simulink model "PLL_complete"  (Simulink 7.7)
settings: Solver=ode45  StartTime=0.0  StopTime=simtime  RelTol=1e-3
values from neighbouring files (symbols this model uses):
  cycles = input('\nNo. of cycles to be observed per change: ')    [PLL_Init_complete.m]
  fq_step = input('Frequency step observed (indicate +/-) (Hz): ')    [PLL_Init_complete.m]
  k = sqrt(2)    [PLL_Init_complete.m]
  ki = (wn^2)/Em    [PLL_Init_complete.m]    (also in plot3D_selfconsistent_cardan_complete.m)
  kp = 2*del*wn/Em    [PLL_Init_complete.m]    (also in plot3D_selfconsistent_cardan_complete.m)
  ph_jump = input('Phase jump observed (indicate +/-) (rad): ')    [PLL_Init_complete.m]
  Ts = 0.1e-3    (= 0.0001)    [PLL_Init_complete.m]
  wc = 2*pi*50    (= 314.159265359)    [PLL_Init_complete.m]
  wf = 2*pi*50/sqrt(2)    [PLL_Init_complete.m]
libraries: aerolibobsolete x7
settings Model: Creator=pradhyumna  LastModifiedBy=Sambhav

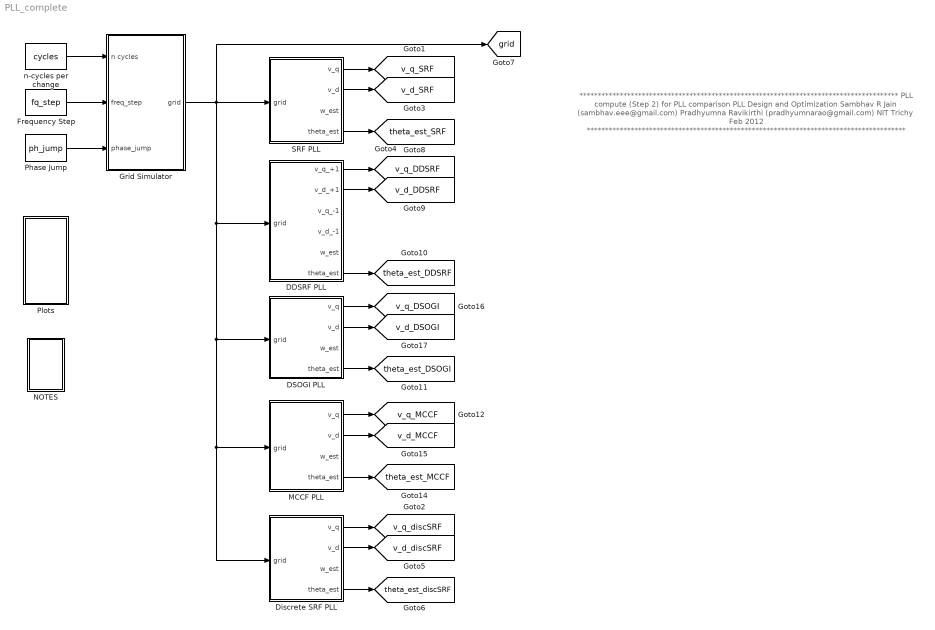
== system PLL_complete ==
  note: ***************************************************************************************
      | PLL compute (Step 2) for PLL comparison
      |
      | PLL Design and Optimization
      |
      | Sambhav R Jain (sambhav.eee@gmail.com)
      | Pradhyumna Ravikirthi (pradhyumnarao@gmail.com)
      | NIT Trichy
      | Feb 2012
      |
      | ***************************************************************************************
  DDSRF PLL : Subsystem
  DSOGI PLL : Subsystem
  Discrete SRF PLL : Subsystem
  Frequency Step : Constant  Value=fq_step
  Grid Simulator : Subsystem
  MCCF PLL : Subsystem
  NOTES : Subsystem
  Phase Jump : Constant  Value=ph_jump
  Plots : Subsystem
  SRF PLL : Subsystem
  n-cycles per change : Constant  Value=cycles
  tag scope: grid=global, theta_est_DDSRF=global, theta_est_DSOGI=global, theta_est_MCCF=global, theta_est_SRF=global, theta_est_discSRF=global, v_d_DDSRF=global, v_d_DSOGI=global, v_d_MCCF=global, v_d_SRF=global, v_d_discSRF=global, v_q_DDSRF=global, v_q_DSOGI=global, v_q_MCCF=global, v_q_SRF=global, v_q_discSRF=global
  wires:
  SRF PLL/1(v_q) -> [v_q_SRF]
  SRF PLL/2(v_d) -> [v_d_SRF]
  SRF PLL/4(theta_est) -> [theta_est_SRF]
  DDSRF PLL/1(v_q_+1) -> [v_q_DDSRF]
  DDSRF PLL/2(v_d_+1) -> [v_d_DDSRF]
  DDSRF PLL/6(theta_est) -> [theta_est_DDSRF]
  DSOGI PLL/1(v_q) -> [v_q_DSOGI]
  DSOGI PLL/2(v_d) -> [v_d_DSOGI]
  DSOGI PLL/4(theta_est) -> [theta_est_DSOGI]
  MCCF PLL/1(v_q) -> [v_q_MCCF]
  MCCF PLL/2(v_d) -> [v_d_MCCF]
  MCCF PLL/4(theta_est) -> [theta_est_MCCF]
  Discrete SRF PLL/1(v_q) -> [v_q_discSRF]
  Discrete SRF PLL/2(v_d) -> [v_d_discSRF]
  Discrete SRF PLL/4(theta_est) -> [theta_est_discSRF]
  n-cycles per change/1 -> Grid Simulator/1(n cycles)
  Frequency Step/1 -> Grid Simulator/2(freq_step)
  Phase Jump/1 -> Grid Simulator/3(phase_jump)
  Grid Simulator/1(grid) -> SRF PLL/1(grid), DDSRF PLL/1(grid), DSOGI PLL/1(grid), MCCF PLL/1(grid), Discrete SRF PLL/1(grid), [grid]

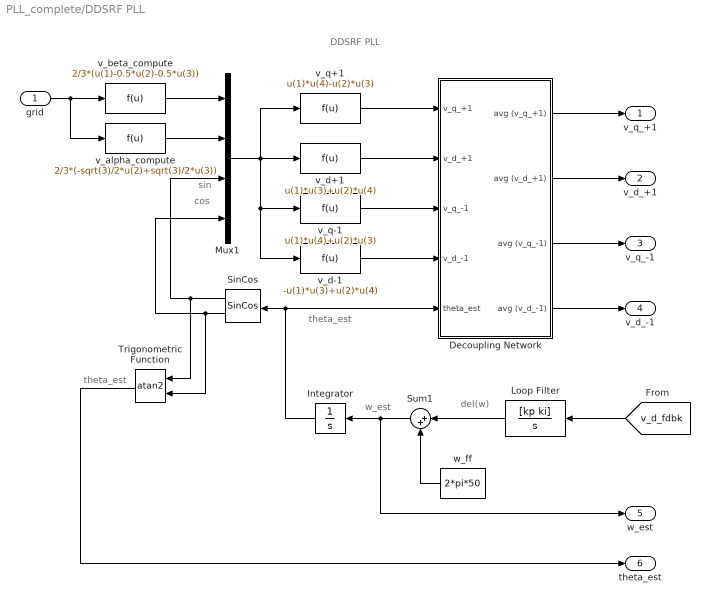
== system PLL_complete/DDSRF PLL ==
  note: cos
  note: sin
  note: del(w)
  note: w_est
  note: theta_est
  note: DDSRF PLL
  note: theta_est
  grid : Inport
  Decoupling Network : Subsystem
  Integrator : Integrator
  Loop Filter : TransferFcn  Numerator=[kp ki]  Denominator=[1 0]
  Mux1 : Mux
  SinCos : aerolibobsolete/SinCos  SystemSampleTime=-1
  Sum1 : Sum  Inputs=|++
  Trigonometric Function : Trigonometry  Operator=atan2
  v_alpha_compute : Fcn  Expr=2/3*(-sqrt(3)/2*u(2)+sqrt(3)/2*u(3))
  v_beta_compute : Fcn  Expr=2/3*(u(1)-0.5*u(2)-0.5*u(3))
  v_d+1 : Fcn  Expr=u(1)*u(3)+u(2)*u(4)
  v_d-1 : Fcn  Expr=-u(1)*u(3)+u(2)*u(4)
  v_q+1 : Fcn  Expr=u(1)*u(4)-u(2)*u(3)
  v_q-1 : Fcn  Expr=u(1)*u(4)+u(2)*u(3)
  w_ff : Constant  Value=2*pi*50
  v_q_+1 : Outport
  v_d_+1 : Outport  Port=2
  v_q_-1 : Outport  Port=3
  v_d_-1 : Outport  Port=4
  w_est : Outport  Port=5
  theta_est : Outport  Port=6
  wires:
  SinCos/2 -> Mux1/4, Trigonometric Function/2
  SinCos/1 -> Mux1/3, Trigonometric Function/1
  v_alpha_compute/1 -> Mux1/2
  v_beta_compute/1 -> Mux1/1
  v_q+1/1 -> Decoupling Network/1(v_q_+1)
  v_d+1/1 -> Decoupling Network/2(v_d_+1)
  v_q-1/1 -> Decoupling Network/3(v_q_-1)
  v_d-1/1 -> Decoupling Network/4(v_d_-1)
  Mux1/1 -> v_d+1/1, v_q+1/1, v_q-1/1, v_d-1/1
  Loop Filter/1 -> Sum1/1
  Sum1/1 -> Integrator/1, w_est/1
  w_ff/1 -> Sum1/2
  Decoupling Network/2(avg (v_d_+1)) -> v_d_+1/1
  Integrator/1 -> SinCos/1, Decoupling Network/5(theta_est)
  grid/1 -> v_beta_compute/1, v_alpha_compute/1
  Decoupling Network/1(avg (v_q_+1)) -> v_q_+1/1
  Trigonometric Function/1 -> theta_est/1
  Decoupling Network/3(avg (v_q_-1)) -> v_q_-1/1
  Decoupling Network/4(avg (v_d_-1)) -> v_d_-1/1
  [v_d_fdbk] -> Loop Filter/1

== system PLL_complete/DSOGI PLL ==
  note: check it out for k = 0.1 !!!!
      | sluggish response
  note: DSOGI PLL
  grid : Inport
  Gain : Gain  Gain=1/2
  Gain1 : Gain  Gain=1/2
  SOGI - alpha : Subsystem
  SOGI - beta : Subsystem
  SRFPLL : Subsystem
  Saturation : Saturate  UpperLimit=2*pi*60  LowerLimit=2*pi*40
  Sum : Sum  Inputs=|++
  Sum1 : Sum  Inputs=|-+
  to reduce  sampling rate of SRF PLL : Gain  SampleTime=0.01
  v_alpha_compute : Fcn  Expr=2/3*(-sqrt(3)/2*u(2)+sqrt(3)/2*u(3))
  v_beta_compute : Fcn  Expr=2/3*(u(1)-0.5*u(2)-0.5*u(3))
  v_q : Outport
  v_d : Outport  Port=2
  w_est : Outport  Port=3
  theta_est : Outport  Port=4
  tag scope: w_est_DSOGI=global
  wires:
  v_alpha_compute/1 -> SOGI - alpha/1(v_alpha)
  v_beta_compute/1 -> SOGI - beta/1(v_beta)
  grid/1 -> v_alpha_compute/1, v_beta_compute/1
  SOGI - beta/1(v_beta_dash) -> Sum/1
  SOGI - alpha/2(q_v_alpha_dash) -> Sum/2
  SOGI - beta/2(q_v_beta_dash) -> Sum1/1
  SOGI - alpha/1(v_alpha_dash) -> Sum1/2
  Sum/1 -> Gain/1
  Gain/1 -> SRFPLL/1(v_beta_1+)
  Sum1/1 -> Gain1/1
  to reduce  sampling rate of SRF PLL/1 -> Saturation/1
  Saturation/1 -> [w_est_DSOGI]
  SRFPLL/4(w_est) -> to reduce  sampling rate of SRF PLL/1, w_est/1
  SRFPLL/1(V_q_space_vector) -> v_q/1
  SRFPLL/2(V_d_error) -> v_d/1
  SRFPLL/3(theta_est) -> theta_est/1
  Gain1/1 -> SRFPLL/2(v_alpha_1+)

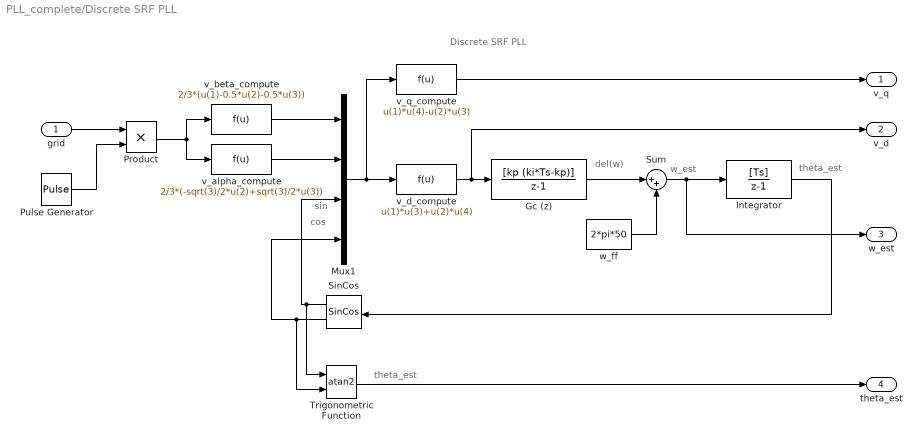
== system PLL_complete/Discrete SRF PLL ==
  note: theta_est
  note: w_est
  note: del(w)
  note: theta_est
  note: Discrete SRF PLL
  note: cos
  note: sin
  grid : Inport
  Gc (z) : DiscreteTransferFcn  Numerator=[kp (ki*Ts-kp)]  Denominator=[1 -1]  SampleTime=0.0001
  Integrator : DiscreteTransferFcn  Numerator=[Ts]  Denominator=[1 -1]  SampleTime=0.0001
  Mux1 : Mux
  Product : Product  RndMeth=Zero
  Pulse Generator : DiscretePulseGenerator  PulseType=Time based  Period=Ts  PulseWidth=10
  SinCos : aerolibobsolete/SinCos  SystemSampleTime=-1
  Sum : Sum  Inputs=|++
  Trigonometric Function : Trigonometry  Operator=atan2
  v_alpha_compute : Fcn  Expr=2/3*(-sqrt(3)/2*u(2)+sqrt(3)/2*u(3))
  v_beta_compute : Fcn  Expr=2/3*(u(1)-0.5*u(2)-0.5*u(3))
  v_d_compute : Fcn  Expr=u(1)*u(3)+u(2)*u(4)
  v_q_compute : Fcn  Expr=u(1)*u(4)-u(2)*u(3)
  w_ff : Constant  Value=2*pi*50
  v_q : Outport
  v_d : Outport  Port=2
  w_est : Outport  Port=3
  theta_est : Outport  Port=4
  wires:
  Trigonometric Function/1 -> theta_est/1
  v_q_compute/1 -> v_q/1
  w_ff/1 -> Sum/2
  v_beta_compute/1 -> Mux1/1
  v_alpha_compute/1 -> Mux1/2
  SinCos/1 -> Trigonometric Function/1, Mux1/3
  SinCos/2 -> Trigonometric Function/2, Mux1/4
  Mux1/1 -> v_q_compute/1, v_d_compute/1
  v_d_compute/1 -> v_d/1, Gc (z)/1
  Sum/1 -> w_est/1, Integrator/1
  Gc (z)/1 -> Sum/1
  Integrator/1 -> SinCos/1
  Pulse Generator/1 -> Product/2
  Product/1 -> v_beta_compute/1, v_alpha_compute/1
  grid/1 -> Product/1

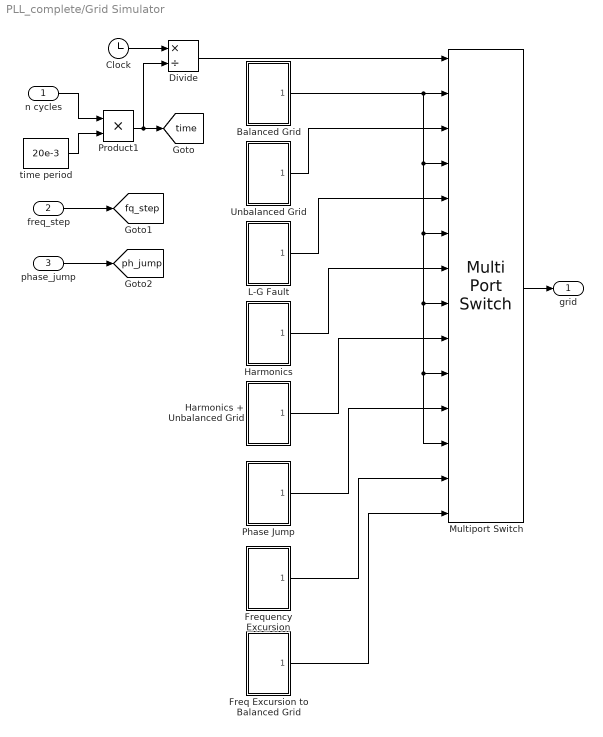
== system PLL_complete/Grid Simulator ==
  n cycles : Inport
  freq_step : Inport  Port=2
  phase_jump : Inport  Port=3
  Balanced Grid : Subsystem
  Clock : Clock
  Divide : Product  Inputs=*/
  Freq Excursion to Balanced Grid : Subsystem
  Frequency Excursion : Subsystem
  Harmonics : Subsystem
  Harmonics + Unbalanced Grid : Subsystem
  L-G Fault : Subsystem
  Multiport Switch : MultiPortSwitch  Inputs=13  DiagnosticForDefault=None  zeroidx=off
  Phase Jump : Subsystem
  Product1 : Product  RndMeth=Zero
  Unbalanced Grid : Subsystem
  time period : Constant  Value=20e-3
  grid : Outport
  tag scope: fq_step=global, ph_jump=global, time=global
  wires:
  Clock/1 -> Divide/1
  time period/1 -> Product1/2
  Product1/1 -> Divide/2, [time]
  Divide/1 -> Multiport Switch/1
  n cycles/1 -> Product1/1
  Multiport Switch/1 -> grid/1
  freq_step/1 -> [fq_step]
  Balanced Grid/1(v_grid) -> Multiport Switch/2, Multiport Switch/4, Multiport Switch/6, Multiport Switch/8, Multiport Switch/10, Multiport Switch/12
  Unbalanced Grid/1(v_grid) -> Multiport Switch/3
  L-G Fault/1(v_grid) -> Multiport Switch/5
  Harmonics/1(v_grid) -> Multiport Switch/7
  Harmonics + Unbalanced Grid/1(v_grid) -> Multiport Switch/9
  phase_jump/1 -> [ph_jump]
  Phase Jump/1(v_grid) -> Multiport Switch/11
  Frequency Excursion/1(v_grid) -> Multiport Switch/13
  Freq Excursion to Balanced Grid/1(v_grid) -> Multiport Switch/14

== system PLL_complete/MCCF PLL ==
  note: MCCF PLL
  grid : Inport
  MCCF module : Subsystem
  SRFPLL : Subsystem
  Saturation : Saturate  UpperLimit=2*pi*60  LowerLimit=2*pi*40
  to reduce  sampling rate of SRF PLL : Gain  SampleTime=0.01
  v_alpha_compute : Fcn  Expr=2/3*(-sqrt(3)/2*u(2)+sqrt(3)/2*u(3))
  v_beta_compute : Fcn  Expr=2/3*(u(1)-0.5*u(2)-0.5*u(3))
  v_q : Outport
  v_d : Outport  Port=2
  w_est : Outport  Port=3
  theta_est : Outport  Port=4
  tag scope: w_est_MCCF=global
  wires:
  v_alpha_compute/1 -> MCCF module/2(v_alpha)
  v_beta_compute/1 -> MCCF module/1(v_beta)
  MCCF module/1(v_beta_est_1+) -> SRFPLL/1(v_beta_1+)
  MCCF module/2(v_alpha_est_1+) -> SRFPLL/2(v_alpha_1+)
  to reduce  sampling rate of SRF PLL/1 -> Saturation/1
  Saturation/1 -> [w_est_MCCF]
  SRFPLL/4(w_est) -> to reduce  sampling rate of SRF PLL/1, w_est/1
  grid/1 -> v_beta_compute/1, v_alpha_compute/1
  SRFPLL/1(V_q_space_vector) -> v_q/1
  SRFPLL/2(V_d_error) -> v_d/1
  SRFPLL/3(theta_est) -> theta_est/1

== system PLL_complete/NOTES ==
  note: T = 0:002247
  note: ki = kp/T
  note: kp = -2.85
  note: Em = - Vm = - 230 * sqrt ( 2 )
      | del = - ( kp / 2 ) * sqrt ( Em / ki )
      | wn = sqrt ( ki * Em )
      | ki = kp / T
  note: Design of kp, ki
      |
      | ki = wn^2 / Em
      | kp = - 2 * del * sqrt ( ki / Em )
      | Weiner Method
      | (for optimum performance)
      | del = 1 / sqrt ( 2 )
  note: Calculated values
      |
      | del = 1 / sqrt ( 2 )
      | wn = 2 * pi * 100
      | ki = - 1213.7
      | kp = - 2.7318
  note: k = 1/sqrt(2) = wf/w
  note: wf = 2*pi*50*k
  note: kp = -20
  note: ki = - 246.7000
  note: Not sure about the loop filter design
  note: DDSRF
  note: k = sqrt(2) ----> optimum performance
  note: DSOGI
  note: MCCF
      | wc = 2*pi*50
  note: plot(time(3500:6500),v_q(3500:6500,:))
  note: k = 0.1 ------> sluggish, but harmonics are dealt well
  note: kp, ki same as DDSRF
  note: k = 1/sqrt(2) = wf/w
  note: wf = 2*pi*50*k
  note: kp = -20
  note: ki = - 246.7000
  note: Not sure about the loop filter design
  note: DDSRF

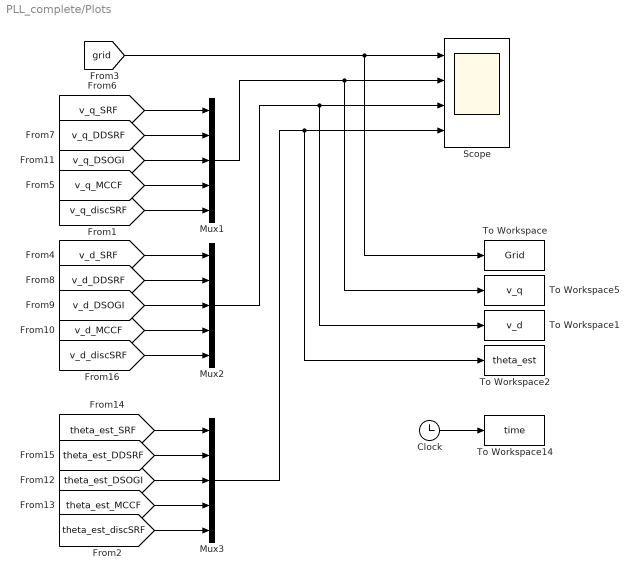
== system PLL_complete/Plots ==
  Clock : Clock
      settings: Decimation=10
  Mux1 : Mux  Inputs=5
  Mux2 : Mux  Inputs=5
  Mux3 : Mux  Inputs=5
  Scope : Scope  NumInputPorts=4
      settings: YMin=-400~-250~-300~-4  YMax=400~350~350~4  SampleInput=on  SampleTime=0.0001
  To Workspace : ToWorkspace  VariableName=Grid  SampleTime=0.0001  SaveFormat=Array
  To Workspace1 : ToWorkspace  VariableName=v_d  SampleTime=0.0001  SaveFormat=Array
  To Workspace14 : ToWorkspace  VariableName=time  SampleTime=0.0001  SaveFormat=Array
  To Workspace2 : ToWorkspace  VariableName=theta_est  SampleTime=0.0001  SaveFormat=Array
  To Workspace5 : ToWorkspace  VariableName=v_q  SampleTime=0.0001  SaveFormat=Array
  wires:
  [grid] -> To Workspace/1, Scope/1
  Clock/1 -> To Workspace14/1
  [v_d_SRF] -> Mux2/1
  [v_d_DDSRF] -> Mux2/2
  [v_d_DSOGI] -> Mux2/3
  [v_d_MCCF] -> Mux2/4
  [v_q_SRF] -> Mux1/1
  [v_q_DDSRF] -> Mux1/2
  [v_q_DSOGI] -> Mux1/3
  [v_q_MCCF] -> Mux1/4
  [theta_est_SRF] -> Mux3/1
  [theta_est_DDSRF] -> Mux3/2
  [theta_est_DSOGI] -> Mux3/3
  [theta_est_MCCF] -> Mux3/4
  Mux1/1 -> To Workspace5/1, Scope/2
  Mux2/1 -> To Workspace1/1, Scope/3
  Mux3/1 -> Scope/4, To Workspace2/1
  [v_q_discSRF] -> Mux1/5
  [v_d_discSRF] -> Mux2/5
  [theta_est_discSRF] -> Mux3/5

== system PLL_complete/SRF PLL ==
  note: sin
  note: cos
  note: SRF PLL
  note: theta_est
  note: del(w)
  note: w_est
  note: theta_est
  grid : Inport
  Integrator : Integrator
  Loop Filter : TransferFcn  Numerator=[kp ki]  Denominator=[1 0]
  Mux1 : Mux
  SinCos : aerolibobsolete/SinCos  SystemSampleTime=-1
  Sum : Sum  Inputs=|++
  Trigonometric Function : Trigonometry  Operator=atan2
  v_alpha_compute : Fcn  Expr=2/3*(-sqrt(3)/2*u(2)+sqrt(3)/2*u(3))
  v_beta_compute : Fcn  Expr=2/3*(u(1)-0.5*u(2)-0.5*u(3))
  v_d_compute : Fcn  Expr=u(1)*u(3)+u(2)*u(4)
  v_q_compute : Fcn  Expr=u(1)*u(4)-u(2)*u(3)
  w_ff : Constant  Value=2*pi*50
  v_q : Outport
  v_d : Outport  Port=2
  w_est : Outport  Port=3
  theta_est : Outport  Port=4
  wires:
  Loop Filter/1 -> Sum/1
  Sum/1 -> Integrator/1, w_est/1
  v_d_compute/1 -> Loop Filter/1, v_d/1
  Integrator/1 -> SinCos/1
  Mux1/1 -> v_d_compute/1, v_q_compute/1
  SinCos/2 -> Mux1/4, Trigonometric Function/2
  SinCos/1 -> Mux1/3, Trigonometric Function/1
  v_alpha_compute/1 -> Mux1/2
  v_beta_compute/1 -> Mux1/1
  grid/1 -> v_beta_compute/1, v_alpha_compute/1
  w_ff/1 -> Sum/2
  v_q_compute/1 -> v_q/1
  Trigonometric Function/1 -> theta_est/1

== system PLL_complete/DDSRF PLL/Decoupling Network ==
  v_q_+1 : Inport
  v_d_+1 : Inport  Port=2
  v_q_-1 : Inport  Port=3
  v_d_-1 : Inport  Port=4
  theta_est : Inport  Port=5
  DC(n/m) +ve : Subsystem
  DC(n/m) -ve : Subsystem
  LPF{1..4} (4 alike) : TransferFcn  Numerator=[wf]  Denominator=[1 wf]
  avg (v_q_+1) : Outport
  avg (v_d_+1) : Outport  Port=2
  avg (v_q_-1) : Outport  Port=3
  avg (v_d_-1) : Outport  Port=4
  tag scope: v_d_fdbk=global
  wires:
  DC(n/m) +ve/1(v_q_+1*) -> LPF1/1
  DC(n/m) +ve/2(v_d_+1*) -> LPF2/1, [v_d_fdbk]
  DC(n/m) -ve/1(v_q_-1*) -> LPF3/1
  DC(n/m) -ve/2(v_d_-1*) -> LPF4/1
  LPF4/1 -> DC(n/m) +ve/2(avg (v_d_-1)), avg (v_d_-1)/1
  LPF3/1 -> DC(n/m) +ve/3(avg (v_q_-1)), avg (v_q_-1)/1
  LPF2/1 -> DC(n/m) -ve/2(avg (v_d_+1)), avg (v_d_+1)/1
  LPF1/1 -> DC(n/m) -ve/3(avg (v_q_+1)), avg (v_q_+1)/1
  theta_est/1 -> DC(n/m) +ve/5(theta_est), DC(n/m) -ve/5(theta_est)
  v_q_+1/1 -> DC(n/m) +ve/1(v_q_+1)
  v_d_+1/1 -> DC(n/m) +ve/4(v_d_+1)
  v_q_-1/1 -> DC(n/m) -ve/1(v_q_-1)
  v_d_-1/1 -> DC(n/m) -ve/4(v_d_-1)

== system PLL_complete/DSOGI PLL/SOGI - alpha ==
  v_alpha : Inport
  Gain : Gain  Gain=k
  Integrator : Integrator
  Integrator1 : Integrator
  Product : Product  RndMeth=Zero
  Product1 : Product  RndMeth=Zero
  Sum : Sum  Inputs=-+|
  Sum1 : Sum  Inputs=|+-
  v_alpha_dash : Outport
  q_v_alpha_dash : Outport  Port=2
  wires:
  v_alpha/1 -> Sum/2
  Product1/1 -> q_v_alpha_dash/1, Sum1/2
  Integrator1/1 -> Product1/1
  Integrator/1 -> v_alpha_dash/1, Integrator1/1, Sum/1
  Product/1 -> Integrator/1
  Sum1/1 -> Product/2
  [w_est_DSOGI] -> Product/1
  Gain/1 -> Sum1/1
  Sum/1 -> Gain/1
  [w_est_DSOGI] -> Product1/2

== system PLL_complete/DSOGI PLL/SOGI - beta ==
  v_beta : Inport
  Gain : Gain  Gain=k
  Integrator : Integrator
  Integrator1 : Integrator
  Product : Product  RndMeth=Zero
  Product1 : Product  RndMeth=Zero
  Sum : Sum  Inputs=-+|
  Sum1 : Sum  Inputs=|+-
  v_beta_dash : Outport
  q_v_beta_dash : Outport  Port=2
  wires:
  Sum/1 -> Gain/1
  Gain/1 -> Sum1/1
  [w_est_DSOGI] -> Product/1
  Sum1/1 -> Product/2
  Product/1 -> Integrator/1
  Integrator/1 -> Sum/1, Integrator1/1, v_beta_dash/1
  Integrator1/1 -> Product1/1
  [w_est_DSOGI] -> Product1/2
  Product1/1 -> Sum1/2, q_v_beta_dash/1
  v_beta/1 -> Sum/2

== system PLL_complete/DSOGI PLL/SRFPLL ==
  note: cos
  note: sin
  note: theta_est
  note: del(w)
  note: w_est
  v_beta_1+ : Inport
  v_alpha_1+ : Inport  Port=2
  Integrator : Integrator
  Loop Filter : TransferFcn  Numerator=[kp ki]  Denominator=[1 0]
  Mux1 : Mux
  SinCos : aerolibobsolete/SinCos  SystemSampleTime=-1
  Sum : Sum  Inputs=|++
  Trigonometric Function : Trigonometry  Operator=atan2
  v_d_compute : Fcn  Expr=u(1)*u(3)+u(2)*u(4)
  v_q_compute : Fcn  Expr=u(1)*u(4)-u(2)*u(3)
  w_ff : Constant  Value=2*pi*50
  V_q_space_vector : Outport
  V_d_error : Outport  Port=2
  theta_est : Outport  Port=3
  w_est : Outport  Port=4
  wires:
  Loop Filter/1 -> Sum/1
  w_ff/1 -> Sum/2
  Sum/1 -> w_est/1, Integrator/1
  v_d_compute/1 -> Loop Filter/1, V_d_error/1
  Integrator/1 -> SinCos/1
  Mux1/1 -> v_d_compute/1, v_q_compute/1
  SinCos/2 -> Mux1/4, Trigonometric Function/2
  SinCos/1 -> Mux1/3, Trigonometric Function/1
  v_beta_1+/1 -> Mux1/1
  v_alpha_1+/1 -> Mux1/2
  v_q_compute/1 -> V_q_space_vector/1
  Trigonometric Function/1 -> theta_est/1

== system PLL_complete/Grid Simulator/Balanced Grid ==
  Mux : Mux  Inputs=3
  v_a : Sin  Amplitude=230*sqrt(2)  Frequency=2*pi*50  Phase=pi/2  SampleTime=0
  v_b : Sin  Amplitude=230*sqrt(2)  Frequency=2*pi*50  Phase=pi/2-2*pi/3  SampleTime=0
  v_c : Sin  Amplitude=230*sqrt(2)  Frequency=2*pi*50  Phase=pi/2+2*pi/3  SampleTime=0
  v_grid : Outport
  wires:
  v_a/1 -> Mux/1
  v_b/1 -> Mux/2
  v_c/1 -> Mux/3
  Mux/1 -> v_grid/1

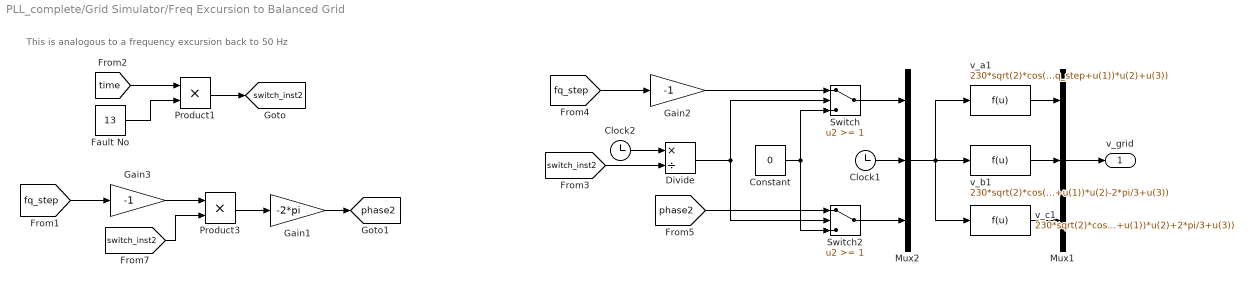
== system PLL_complete/Grid Simulator/Freq Excursion to Balanced Grid ==
  note: This is analogous to a frequency excursion back to 50 Hz
  Clock1 : Clock
      settings: Decimation=10
  Clock2 : Clock
      settings: Decimation=10
  Constant : Constant  Value=0
  Divide : Product  Inputs=*/
  Fault No : Constant  Value=13
  Gain1 : Gain  Gain=-2*pi
  Gain2 : Gain  Gain=-1
  Gain3 : Gain  Gain=-1
  Mux1 : Mux  Inputs=3
  Mux2 : Mux  Inputs=3
  Product1 : Product  RndMeth=Zero
  Product3 : Product  RndMeth=Zero
  Switch : Switch  Threshold=1
  Switch2 : Switch  Threshold=1
  v_a1 : Fcn  Expr=230*sqrt(2)*cos(2*pi*(50+fq_step+u(1))*u(2)+u(3))
  v_b1 : Fcn  Expr=230*sqrt(2)*cos(2*pi*(50+fq_step+u(1))*u(2)-2*pi/3+u(3))
  v_c1 : Fcn  Expr=230*sqrt(2)*cos(2*pi*(50+fq_step+u(1))*u(2)+2*pi/3+u(3))
  v_grid : Outport
  tag scope: phase2=global, switch_inst2=global
  wires:
  Gain1/1 -> [phase2]
  Product3/1 -> Gain1/1
  [switch_inst2] -> Product3/2
  Product1/1 -> [switch_inst2]
  Fault No/1 -> Product1/2
  [time] -> Product1/1
  [phase2] -> Switch2/1
  Constant/1 -> Switch2/3, Switch/3
  Clock1/1 -> Mux2/2
  Divide/1 -> Switch2/2, Switch/2
  [switch_inst2] -> Divide/2
  Clock2/1 -> Divide/1
  Switch/1 -> Mux2/1
  Mux1/1 -> v_grid/1
  Switch2/1 -> Mux2/3
  v_c1/1 -> Mux1/3
  v_b1/1 -> Mux1/2
  v_a1/1 -> Mux1/1
  Mux2/1 -> v_c1/1, v_b1/1, v_a1/1
  Gain2/1 -> Switch/1
  [fq_step] -> Gain2/1
  Gain3/1 -> Product3/1
  [fq_step] -> Gain3/1

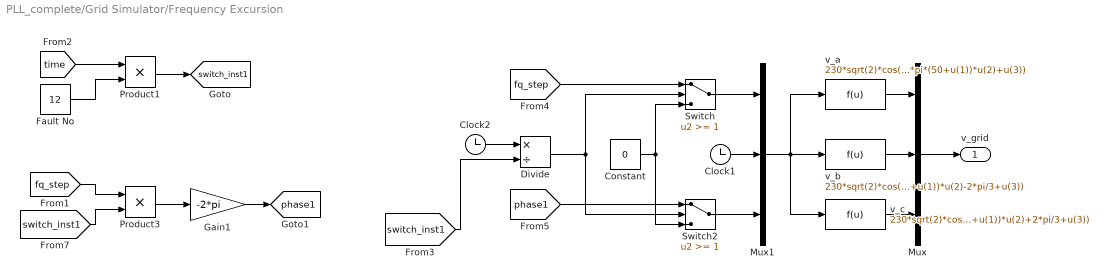
== system PLL_complete/Grid Simulator/Frequency Excursion ==
  Clock1 : Clock
      settings: Decimation=10
  Clock2 : Clock
      settings: Decimation=10
  Constant : Constant  Value=0
  Divide : Product  Inputs=*/
  Fault No : Constant  Value=12
  Gain1 : Gain  Gain=-2*pi
  Mux : Mux  Inputs=3
  Mux1 : Mux  Inputs=3
  Product1 : Product  RndMeth=Zero
  Product3 : Product  RndMeth=Zero
  Switch : Switch  Threshold=1
  Switch2 : Switch  Threshold=1
  v_a : Fcn  Expr=230*sqrt(2)*cos(2*pi*(50+u(1))*u(2)+u(3))
  v_b : Fcn  Expr=230*sqrt(2)*cos(2*pi*(50+u(1))*u(2)-2*pi/3+u(3))
  v_c : Fcn  Expr=230*sqrt(2)*cos(2*pi*(50+u(1))*u(2)+2*pi/3+u(3))
  v_grid : Outport
  tag scope: phase1=global, switch_inst1=global
  wires:
  [phase1] -> Switch2/1
  Gain1/1 -> [phase1]
  Constant/1 -> Switch2/3, Switch/3
  Product3/1 -> Gain1/1
  [switch_inst1] -> Product3/2
  [fq_step] -> Product3/1
  Product1/1 -> [switch_inst1]
  Clock1/1 -> Mux1/2
  Divide/1 -> Switch2/2, Switch/2
  [switch_inst1] -> Divide/2
  Clock2/1 -> Divide/1
  Switch/1 -> Mux1/1
  Mux/1 -> v_grid/1
  Fault No/1 -> Product1/2
  [time] -> Product1/1
  Switch2/1 -> Mux1/3
  v_c/1 -> Mux/3
  v_b/1 -> Mux/2
  v_a/1 -> Mux/1
  Mux1/1 -> v_c/1, v_b/1, v_a/1
  [fq_step] -> Switch/1

== system PLL_complete/Grid Simulator/Harmonics ==
  Harmonics Generator : Subsystem
  Mux : Mux  Inputs=3
  v_grid : Outport
  wires:
  Harmonics Generator/3(v_c) -> Mux/3
  Harmonics Generator/2(v_b) -> Mux/2
  Harmonics Generator/1(v_a) -> Mux/1
  Mux/1 -> v_grid/1

== system PLL_complete/Grid Simulator/Harmonics + Unbalanced Grid ==
  Harmonics + Unbalance  Generator : Subsystem
  Mux1 : Mux  Inputs=3
  v_grid : Outport
  wires:
  Harmonics + Unbalance  Generator/3(v_c) -> Mux1/3
  Harmonics + Unbalance  Generator/2(v_b) -> Mux1/2
  Harmonics + Unbalance  Generator/1(v_a) -> Mux1/1
  Mux1/1 -> v_grid/1

== system PLL_complete/Grid Simulator/L-G Fault ==
  Mux : Mux  Inputs=3
  v_a : Sin  Amplitude=230*sqrt(2)  Frequency=2*pi*50  Phase=pi/2  SampleTime=0
  v_b : Sin  Amplitude=10  Frequency=2*pi*50  Phase=pi/2-2*pi/3  SampleTime=0
  v_c : Sin  Amplitude=230*sqrt(2)  Frequency=2*pi*50  Phase=pi/2+2*pi/3  SampleTime=0
  v_grid : Outport
  wires:
  Mux/1 -> v_grid/1
  v_c/1 -> Mux/3
  v_b/1 -> Mux/2
  v_a/1 -> Mux/1

== system PLL_complete/Grid Simulator/Phase Jump ==
  Clock1 : Clock
      settings: Decimation=10
  Clock2 : Clock
      settings: Decimation=10
  Constant : Constant  Value=0
  Divide : Product  Inputs=*/
  Fault No : Constant  Value=10
  Mux : Mux  Inputs=3
  Mux1 : Mux  Inputs=2
  Product1 : Product  RndMeth=Zero
  Switch : Switch  Threshold=1
  v_a : Fcn  Expr=230*sqrt(2)*cos(2*pi*50*u(1)+u(2))
  v_b : Fcn  Expr=230*sqrt(2)*cos(2*pi*50*u(1)-2*pi/3+u(2))
  v_c : Fcn  Expr=230*sqrt(2)*cos(2*pi*50*u(1)+2*pi/3+u(2))
  v_grid : Outport
  tag scope: switch_inst3=global
  wires:
  Constant/1 -> Switch/3
  Product1/1 -> [switch_inst3]
  Divide/1 -> Switch/2
  [switch_inst3] -> Divide/2
  Clock2/1 -> Divide/1
  Mux/1 -> v_grid/1
  Fault No/1 -> Product1/2
  [time] -> Product1/1
  v_c/1 -> Mux/3
  v_b/1 -> Mux/2
  v_a/1 -> Mux/1
  Mux1/1 -> v_c/1, v_b/1, v_a/1
  [ph_jump] -> Switch/1
  Clock1/1 -> Mux1/1
  Switch/1 -> Mux1/2

== system PLL_complete/Grid Simulator/Unbalanced Grid ==
  Mux : Mux  Inputs=3
  v_a : Sin  Amplitude=230*sqrt(2)  Frequency=2*pi*50  Phase=pi/2  SampleTime=0
  v_b : Sin  Amplitude=200*sqrt(2)  Frequency=2*pi*50  Phase=pi/2-2*pi/3  SampleTime=0
  v_c : Sin  Amplitude=210*sqrt(2)  Frequency=2*pi*50  Phase=pi/2+2*pi/3  SampleTime=0
  v_grid : Outport
  wires:
  v_a/1 -> Mux/1
  v_b/1 -> Mux/2
  v_c/1 -> Mux/3
  Mux/1 -> v_grid/1

== system PLL_complete/MCCF PLL/MCCF module ==
  v_beta : Inport
  v_alpha : Inport  Port=2
  Subsystem : Subsystem
  Sum : Sum  Inputs=|+-
  Sum1 : Sum  Inputs=|+-
  Sum2 : Sum  Inputs=+|+|+|+|+|+|+|+
  Sum6 : Sum  Inputs=+|+|+|+|+|+|+|+
  v_beta_est_1+ : Outport
  v_alpha_est_1+ : Outport  Port=2
  v_beta_est_1- : Outport  Port=3
  v_alpha_est_1- : Outport  Port=4
  wires:
  Sum2/1 -> Sum1/2
  Sum6/1 -> Sum/2
  Subsystem/16(v_alpha_est_11-) -> Sum2/8
  Subsystem/14(v_alpha_est_11+) -> Sum2/7
  Subsystem/12(v_alpha_est_7-) -> Sum2/6
  Subsystem/10(v_alpha_est_7+) -> Sum2/5
  Subsystem/8(v_alpha_est_5-) -> Sum2/4
  Subsystem/6(v_alpha_est_5+) -> Sum2/3
  Subsystem/4(v_alpha_est_1-) -> Sum2/2, v_alpha_est_1-/1
  Subsystem/2(v_alpha_est_1+) -> Sum2/1, v_alpha_est_1+/1
  Subsystem/15(v_beta_est_11-) -> Sum6/8
  Subsystem/13(v_beta_est_11+) -> Sum6/7
  Subsystem/11(v_beta_est_7-) -> Sum6/6
  Subsystem/9(v_beta_est_7+) -> Sum6/5
  Subsystem/7(v_beta_est_5-) -> Sum6/4
  Subsystem/5(v_beta_est_5+) -> Sum6/3
  Subsystem/3(v_beta_est_1-) -> Sum6/2, v_beta_est_1-/1
  Subsystem/1(v_beta_est_1+) -> Sum6/1, v_beta_est_1+/1
  Sum1/1 -> Subsystem/2(v_alpha_n)
  Sum/1 -> Subsystem/1(v_beta_n)
  v_beta/1 -> Sum/1
  v_alpha/1 -> Sum1/1

== system PLL_complete/MCCF PLL/SRFPLL ==
  note: cos
  note: sin
  note: theta_est
  note: del(w)
  note: w_est
  v_beta_1+ : Inport
  v_alpha_1+ : Inport  Port=2
  Integrator : Integrator
  Loop Filter : TransferFcn  Numerator=[kp ki]  Denominator=[1 0]
  Mux1 : Mux
  SinCos : aerolibobsolete/SinCos  SystemSampleTime=-1
  Sum : Sum  Inputs=|++
  Trigonometric Function : Trigonometry  Operator=atan2
  v_d_compute : Fcn  Expr=u(1)*u(3)+u(2)*u(4)
  v_q_compute : Fcn  Expr=u(1)*u(4)-u(2)*u(3)
  w_ff : Constant  Value=2*pi*50
  V_q_space_vector : Outport
  V_d_error : Outport  Port=2
  theta_est : Outport  Port=3
  w_est : Outport  Port=4
  wires:
  Loop Filter/1 -> Sum/1
  Sum/1 -> Integrator/1, w_est/1
  v_d_compute/1 -> Loop Filter/1, V_d_error/1
  Integrator/1 -> SinCos/1
  Mux1/1 -> v_d_compute/1, v_q_compute/1
  SinCos/2 -> Mux1/4, Trigonometric Function/2
  SinCos/1 -> Mux1/3, Trigonometric Function/1
  v_beta_1+/1 -> Mux1/1
  v_alpha_1+/1 -> Mux1/2
  v_q_compute/1 -> V_q_space_vector/1
  Trigonometric Function/1 -> theta_est/1
  w_ff/1 -> Sum/2

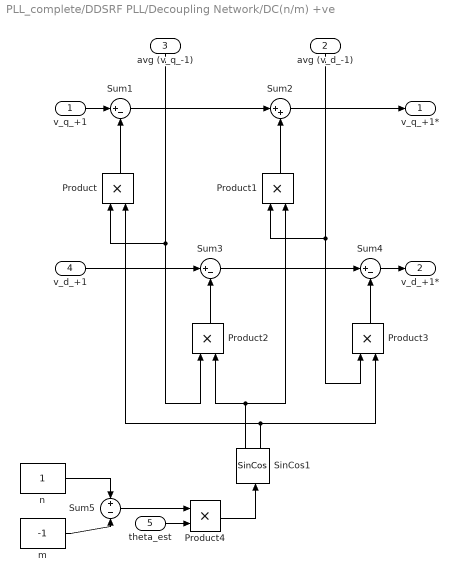
== system PLL_complete/DDSRF PLL/Decoupling Network/DC(n/m) +ve ==
  v_q_+1 : Inport
  avg (v_d_-1) : Inport  Port=2
  avg (v_q_-1) : Inport  Port=3
  v_d_+1 : Inport  Port=4
  theta_est : Inport  Port=5
  Product{,1..4} (5 alike) : Product  RndMeth=Zero
  SinCos1 : aerolibobsolete/SinCos  SystemSampleTime=-1
  Sum1 : Sum  Inputs=|+-
  Sum2 : Sum  Inputs=|++
  Sum3 : Sum  Inputs=|+-
  Sum4 : Sum  Inputs=|+-
  Sum5 : Sum  Inputs=+|-
  m : Constant  Value=-1
  n : Constant
  v_q_+1* : Outport
  v_d_+1* : Outport  Port=2
  wires:
  Product/1 -> Sum1/2
  SinCos1/2 -> Product/2, Product3/2
  Sum1/1 -> Sum2/1
  Product1/1 -> Sum2/2
  SinCos1/1 -> Product1/2, Product2/2
  Product2/1 -> Sum3/2
  Sum3/1 -> Sum4/1
  Product3/1 -> Sum4/2
  avg (v_q_-1)/1 -> Product/1, Product2/1
  avg (v_d_-1)/1 -> Product1/1, Product3/1
  n/1 -> Sum5/1
  Sum5/1 -> Product4/1
  Product4/1 -> SinCos1/1
  m/1 -> Sum5/2
  v_q_+1/1 -> Sum1/1
  Sum2/1 -> v_q_+1*/1
  v_d_+1/1 -> Sum3/1
  Sum4/1 -> v_d_+1*/1
  theta_est/1 -> Product4/2

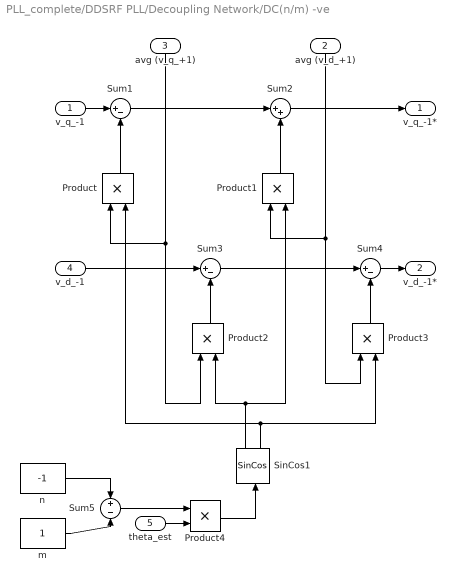
== system PLL_complete/DDSRF PLL/Decoupling Network/DC(n/m) -ve ==
  v_q_-1 : Inport
  avg (v_d_+1) : Inport  Port=2
  avg (v_q_+1) : Inport  Port=3
  v_d_-1 : Inport  Port=4
  theta_est : Inport  Port=5
  Product{,1..4} (5 alike) : Product  RndMeth=Zero
  SinCos1 : aerolibobsolete/SinCos  SystemSampleTime=-1
  Sum1 : Sum  Inputs=|+-
  Sum2 : Sum  Inputs=|++
  Sum3 : Sum  Inputs=|+-
  Sum4 : Sum  Inputs=|+-
  Sum5 : Sum  Inputs=+|-
  m : Constant
  n : Constant  Value=-1
  v_q_-1* : Outport
  v_d_-1* : Outport  Port=2
  wires:
  theta_est/1 -> Product4/2
  Sum4/1 -> v_d_-1*/1
  v_d_-1/1 -> Sum3/1
  Sum2/1 -> v_q_-1*/1
  v_q_-1/1 -> Sum1/1
  m/1 -> Sum5/2
  Product4/1 -> SinCos1/1
  Sum5/1 -> Product4/1
  n/1 -> Sum5/1
  avg (v_d_+1)/1 -> Product3/1, Product1/1
  avg (v_q_+1)/1 -> Product2/1, Product/1
  Product3/1 -> Sum4/2
  Sum3/1 -> Sum4/1
  Product2/1 -> Sum3/2
  SinCos1/1 -> Product2/2, Product1/2
  Product1/1 -> Sum2/2
  Sum1/1 -> Sum2/1
  SinCos1/2 -> Product3/2, Product/2
  Product/1 -> Sum1/2

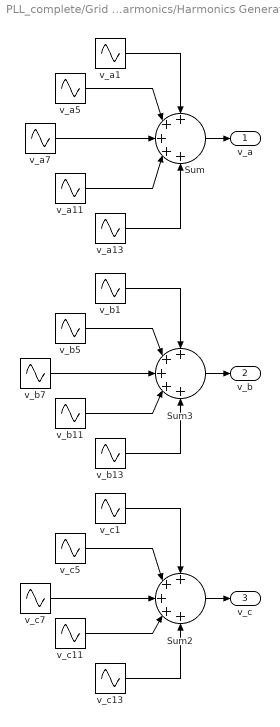
== system PLL_complete/Grid Simulator/Harmonics/Harmonics Generator ==
  Sum : Sum  Inputs=+|+|+|+|+
  Sum2 : Sum  Inputs=+|+|+|+|+
  Sum3 : Sum  Inputs=+|+|+|+|+
  v_a1 : Sin  Amplitude=230*sqrt(2)  Frequency=2*pi*50  Phase=pi/2  SampleTime=0
  v_a11 : Sin  Amplitude=230*sqrt(2)/11/4  Frequency=2*pi*50*11  Phase=pi/2  SampleTime=0
  v_a13 : Sin  Amplitude=230*sqrt(2)/13/4  Frequency=2*pi*50*13  Phase=pi/2  SampleTime=0
  v_a5 : Sin  Amplitude=230*sqrt(2)/5/4  Frequency=2*pi*50*5  Phase=pi/2  SampleTime=0
  v_a7 : Sin  Amplitude=230*sqrt(2)/7/4  Frequency=2*pi*50*7  Phase=pi/2  SampleTime=0
  v_b1 : Sin  Amplitude=230*sqrt(2)  Frequency=2*pi*50  Phase=pi/2-2*pi/3  SampleTime=0
  v_b11 : Sin  Amplitude=230*sqrt(2)/11/4  Frequency=2*pi*50*11  Phase=pi/2-2*pi/3*11  SampleTime=0
  v_b13 : Sin  Amplitude=230*sqrt(2)/13/4  Frequency=2*pi*50*13  Phase=pi/2-2*pi/3*13  SampleTime=0
  v_b5 : Sin  Amplitude=230*sqrt(2)/5/4  Frequency=2*pi*50*5  Phase=pi/2-2*pi/3*5  SampleTime=0
  v_b7 : Sin  Amplitude=230*sqrt(2)/7/4  Frequency=2*pi*50*7  Phase=pi/2-2*pi/3*7  SampleTime=0
  v_c1 : Sin  Amplitude=230*sqrt(2)  Frequency=2*pi*50  Phase=pi/2+2*pi/3  SampleTime=0
  v_c11 : Sin  Amplitude=230*sqrt(2)/11/4  Frequency=2*pi*50*11  Phase=pi/2+2*pi/3*11  SampleTime=0
  v_c13 : Sin  Amplitude=230*sqrt(2)/13/4  Frequency=2*pi*50*13  Phase=pi/2+2*pi/3*13  SampleTime=0
  v_c5 : Sin  Amplitude=230*sqrt(2)/5/4  Frequency=2*pi*50*5  Phase=pi/2+2*pi/3*5  SampleTime=0
  v_c7 : Sin  Amplitude=230*sqrt(2)/7/4  Frequency=2*pi*50*7  Phase=pi/2+2*pi/3*7  SampleTime=0
  v_a : Outport
  v_b : Outport  Port=2
  v_c : Outport  Port=3
  wires:
  Sum2/1 -> v_c/1
  Sum3/1 -> v_b/1
  Sum/1 -> v_a/1
  v_a1/1 -> Sum/1
  v_a5/1 -> Sum/2
  v_a7/1 -> Sum/3
  v_a11/1 -> Sum/4
  v_a13/1 -> Sum/5
  v_b1/1 -> Sum3/1
  v_b5/1 -> Sum3/2
  v_b7/1 -> Sum3/3
  v_b11/1 -> Sum3/4
  v_b13/1 -> Sum3/5
  v_c7/1 -> Sum2/3
  v_c1/1 -> Sum2/1
  v_c5/1 -> Sum2/2
  v_c11/1 -> Sum2/4
  v_c13/1 -> Sum2/5

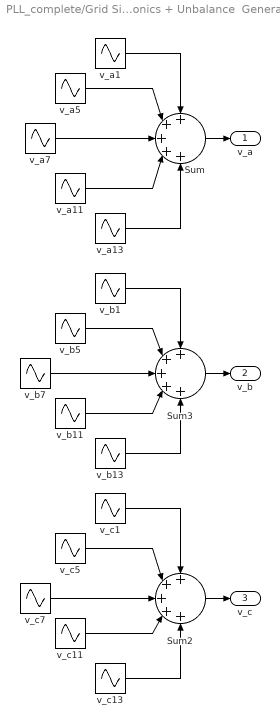
== system PLL_complete/Grid Simulator/Harmonics + Unbalanced Grid/Harmonics + Unbalance  Generator ==
  Sum : Sum  Inputs=+|+|+|+|+
  Sum2 : Sum  Inputs=+|+|+|+|+
  Sum3 : Sum  Inputs=+|+|+|+|+
  v_a1 : Sin  Amplitude=230*sqrt(2)  Frequency=2*pi*50  Phase=pi/2  SampleTime=0
  v_a11 : Sin  Amplitude=230*sqrt(2)/11/4  Frequency=2*pi*50*11  Phase=pi/2  SampleTime=0
  v_a13 : Sin  Amplitude=230*sqrt(2)/13/4  Frequency=2*pi*50*13  Phase=pi/2  SampleTime=0
  v_a5 : Sin  Amplitude=230*sqrt(2)/5/4  Frequency=2*pi*50*5  Phase=pi/2  SampleTime=0
  v_a7 : Sin  Amplitude=230*sqrt(2)/7/4  Frequency=2*pi*50*7  Phase=pi/2  SampleTime=0
  v_b1 : Sin  Amplitude=200*sqrt(2)  Frequency=2*pi*50  Phase=pi/2-2*pi/3+pi/6  SampleTime=0
  v_b11 : Sin  Amplitude=200*sqrt(2)/11/4  Frequency=2*pi*50*11  Phase=pi/2-2*pi/3*11+pi/6*11  SampleTime=0
  v_b13 : Sin  Amplitude=200*sqrt(2)/13/4  Frequency=2*pi*50*13  Phase=pi/2-2*pi/3*13+pi/6*13  SampleTime=0
  v_b5 : Sin  Amplitude=200*sqrt(2)/5/4  Frequency=2*pi*50*5  Phase=pi/2-2*pi/3*5+pi/6*5  SampleTime=0
  v_b7 : Sin  Amplitude=200*sqrt(2)/7/4  Frequency=2*pi*50*7  Phase=pi/2-2*pi/3*7+pi/6*7  SampleTime=0
  v_c1 : Sin  Amplitude=210*sqrt(2)  Frequency=2*pi*50  Phase=pi/2+2*pi/3-pi/18  SampleTime=0
  v_c11 : Sin  Amplitude=210*sqrt(2)/11/4  Frequency=2*pi*50*11  Phase=pi/2+2*pi/3*11-pi/18*11  SampleTime=0
  v_c13 : Sin  Amplitude=210*sqrt(2)/13/4  Frequency=2*pi*50*13  Phase=pi/2+2*pi/3*13-pi/18*13  SampleTime=0
  v_c5 : Sin  Amplitude=210*sqrt(2)/5/4  Frequency=2*pi*50*5  Phase=pi/2+2*pi/3*5-pi/18*5  SampleTime=0
  v_c7 : Sin  Amplitude=210*sqrt(2)/7/4  Frequency=2*pi*50*7  Phase=pi/2+2*pi/3*7-pi/18*7  SampleTime=0
  v_a : Outport
  v_b : Outport  Port=2
  v_c : Outport  Port=3
  wires:
  Sum2/1 -> v_c/1
  Sum3/1 -> v_b/1
  Sum/1 -> v_a/1
  v_a1/1 -> Sum/1
  v_a5/1 -> Sum/2
  v_a7/1 -> Sum/3
  v_a11/1 -> Sum/4
  v_a13/1 -> Sum/5
  v_b1/1 -> Sum3/1
  v_b5/1 -> Sum3/2
  v_b7/1 -> Sum3/3
  v_b11/1 -> Sum3/4
  v_b13/1 -> Sum3/5
  v_c7/1 -> Sum2/3
  v_c1/1 -> Sum2/1
  v_c5/1 -> Sum2/2
  v_c11/1 -> Sum2/4
  v_c13/1 -> Sum2/5

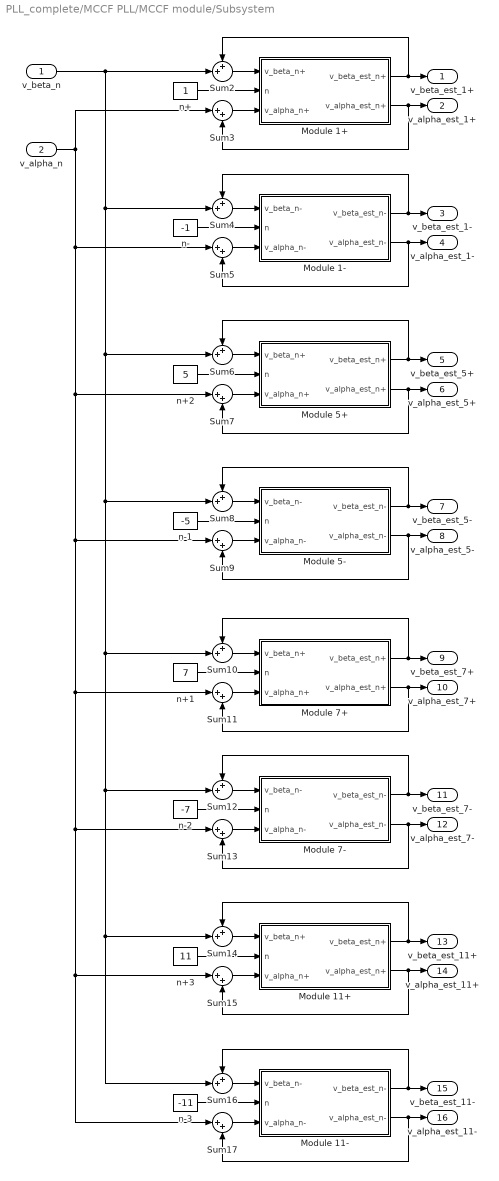
== system PLL_complete/MCCF PLL/MCCF module/Subsystem ==
  v_beta_n : Inport
  v_alpha_n : Inport  Port=2
  Module 1+ : Subsystem
  Module 1- : Subsystem
  Module 11+ : Subsystem
  Module 11- : Subsystem
  Module 5+ : Subsystem
  Module 5- : Subsystem
  Module 7+ : Subsystem
  Module 7- : Subsystem
  Sum{2,4,6,8,10,12,14,16} (8 alike) : Sum  Inputs=++|
  Sum{3,5,7,9,11,13,15,17} (8 alike) : Sum  Inputs=|++
  n+ : Constant
  n+1 : Constant  Value=7
  n+2 : Constant  Value=5
  n+3 : Constant  Value=11
  n- : Constant  Value=-1
  n-1 : Constant  Value=-5
  n-2 : Constant  Value=-7
  n-3 : Constant  Value=-11
  v_beta_est_1+ : Outport
  v_alpha_est_1+ : Outport  Port=2
  v_beta_est_1- : Outport  Port=3
  v_alpha_est_1- : Outport  Port=4
  v_beta_est_5+ : Outport  Port=5
  v_alpha_est_5+ : Outport  Port=6
  v_beta_est_5- : Outport  Port=7
  v_alpha_est_5- : Outport  Port=8
  v_beta_est_7+ : Outport  Port=9
  v_alpha_est_7+ : Outport  Port=10
  v_beta_est_7- : Outport  Port=11
  v_alpha_est_7- : Outport  Port=12
  v_beta_est_11+ : Outport  Port=13
  v_alpha_est_11+ : Outport  Port=14
  v_beta_est_11- : Outport  Port=15
  v_alpha_est_11- : Outport  Port=16
  wires:
  n+/1 -> Module 1+/2(n)
  Sum2/1 -> Module 1+/1(v_beta_n+)
  Sum3/1 -> Module 1+/3(v_alpha_n+)
  Module 1+/1(v_beta_est_n+) -> Sum2/1, v_beta_est_1+/1
  Module 1+/2(v_alpha_est_n+) -> Sum3/2, v_alpha_est_1+/1
  n-/1 -> Module 1-/2(n)
  Sum4/1 -> Module 1-/1(v_beta_n-)
  Sum5/1 -> Module 1-/3(v_alpha_n-)
  Module 1-/1(v_beta_est_n-) -> Sum4/1, v_beta_est_1-/1
  Module 1-/2(v_alpha_est_n-) -> Sum5/2, v_alpha_est_1-/1
  n+2/1 -> Module 5+/2(n)
  Sum6/1 -> Module 5+/1(v_beta_n+)
  Sum7/1 -> Module 5+/3(v_alpha_n+)
  Module 5+/1(v_beta_est_n+) -> Sum6/1, v_beta_est_5+/1
  Module 5+/2(v_alpha_est_n+) -> Sum7/2, v_alpha_est_5+/1
  n-1/1 -> Module 5-/2(n)
  Sum8/1 -> Module 5-/1(v_beta_n-)
  Sum9/1 -> Module 5-/3(v_alpha_n-)
  Module 5-/1(v_beta_est_n-) -> Sum8/1, v_beta_est_5-/1
  Module 5-/2(v_alpha_est_n-) -> Sum9/2, v_alpha_est_5-/1
  n+1/1 -> Module 7+/2(n)
  Sum10/1 -> Module 7+/1(v_beta_n+)
  Sum11/1 -> Module 7+/3(v_alpha_n+)
  Module 7+/1(v_beta_est_n+) -> Sum10/1, v_beta_est_7+/1
  Module 7+/2(v_alpha_est_n+) -> Sum11/2, v_alpha_est_7+/1
  n-2/1 -> Module 7-/2(n)
  Sum12/1 -> Module 7-/1(v_beta_n-)
  Sum13/1 -> Module 7-/3(v_alpha_n-)
  Module 7-/1(v_beta_est_n-) -> Sum12/1, v_beta_est_7-/1
  Module 7-/2(v_alpha_est_n-) -> Sum13/2, v_alpha_est_7-/1
  n+3/1 -> Module 11+/2(n)
  Sum14/1 -> Module 11+/1(v_beta_n+)
  Sum15/1 -> Module 11+/3(v_alpha_n+)
  Module 11+/1(v_beta_est_n+) -> Sum14/1, v_beta_est_11+/1
  Module 11+/2(v_alpha_est_n+) -> Sum15/2, v_alpha_est_11+/1
  n-3/1 -> Module 11-/2(n)
  Sum16/1 -> Module 11-/1(v_beta_n-)
  Sum17/1 -> Module 11-/3(v_alpha_n-)
  Module 11-/1(v_beta_est_n-) -> Sum16/1, v_beta_est_11-/1
  Module 11-/2(v_alpha_est_n-) -> Sum17/2, v_alpha_est_11-/1
  v_beta_n/1 -> Sum16/2, Sum14/2, Sum12/2, Sum10/2, Sum8/2, Sum6/2, Sum4/2, Sum2/2
  v_alpha_n/1 -> Sum17/1, Sum15/1, Sum13/1, Sum11/1, Sum9/1, Sum7/1, Sum5/1, Sum3/1

== system PLL_complete/MCCF PLL/MCCF module/Subsystem/Module 1+ ==
  v_beta_n+ : Inport
  n : Inport  Port=2
  v_alpha_n+ : Inport  Port=3
  Gain{,3..5} (4 alike) : Gain  Gain=wc
  Integrator : Integrator
  Integrator1 : Integrator
  Product : Product  Inputs=3  RndMeth=Zero
  Product2 : Product  Inputs=3  RndMeth=Zero
  Sum : Sum  Inputs=-|+|+
  Sum1 : Sum  Inputs=-|+|-
  v_beta_est_n+ : Outport
  v_alpha_est_n+ : Outport  Port=2
  wires:
  Gain3/1 -> Sum1/3
  Gain/1 -> Sum/1
  Gain4/1 -> Sum/2
  Gain5/1 -> Sum1/2
  Sum1/1 -> Integrator1/1
  Sum/1 -> Integrator/1
  Integrator1/1 -> Gain3/1, v_alpha_est_n+/1, Product/3
  Integrator/1 -> Gain/1, v_beta_est_n+/1, Product2/3
  Product/1 -> Sum/3
  Product2/1 -> Sum1/1
  n/1 -> Product/1, Product2/1
  v_beta_n+/1 -> Gain4/1
  v_alpha_n+/1 -> Gain5/1
  [w_est_MCCF] -> Product/2, Product2/2

== system PLL_complete/MCCF PLL/MCCF module/Subsystem/Module 1- ==
  v_beta_n- : Inport
  n : Inport  Port=2
  v_alpha_n- : Inport  Port=3
  Gain{,3..5} (4 alike) : Gain  Gain=wc
  Integrator : Integrator
  Integrator1 : Integrator
  Product : Product  Inputs=3  RndMeth=Zero
  Product2 : Product  Inputs=3  RndMeth=Zero
  Sum : Sum  Inputs=-|+|+
  Sum1 : Sum  Inputs=-|+|-
  v_beta_est_n- : Outport
  v_alpha_est_n- : Outport  Port=2
  wires:
  [w_est_MCCF] -> Product2/2, Product/2
  v_alpha_n-/1 -> Gain5/1
  v_beta_n-/1 -> Gain4/1
  n/1 -> Product2/1, Product/1
  Product2/1 -> Sum1/1
  Product/1 -> Sum/3
  Integrator/1 -> Product2/3, v_beta_est_n-/1, Gain/1
  Integrator1/1 -> Product/3, v_alpha_est_n-/1, Gain3/1
  Sum/1 -> Integrator/1
  Sum1/1 -> Integrator1/1
  Gain5/1 -> Sum1/2
  Gain4/1 -> Sum/2
  Gain/1 -> Sum/1
  Gain3/1 -> Sum1/3

== system PLL_complete/MCCF PLL/MCCF module/Subsystem/Module 11+ ==
  v_beta_n+ : Inport
  n : Inport  Port=2
  v_alpha_n+ : Inport  Port=3
  Gain{,3..5} (4 alike) : Gain  Gain=wc
  Integrator : Integrator
  Integrator1 : Integrator
  Product : Product  Inputs=3  RndMeth=Zero
  Product2 : Product  Inputs=3  RndMeth=Zero
  Sum : Sum  Inputs=-|+|+
  Sum1 : Sum  Inputs=-|+|-
  v_beta_est_n+ : Outport
  v_alpha_est_n+ : Outport  Port=2
  wires:
  [w_est_MCCF] -> Product2/2, Product/2
  v_alpha_n+/1 -> Gain5/1
  v_beta_n+/1 -> Gain4/1
  n/1 -> Product2/1, Product/1
  Product2/1 -> Sum1/1
  Product/1 -> Sum/3
  Integrator/1 -> Product2/3, v_beta_est_n+/1, Gain/1
  Integrator1/1 -> Product/3, v_alpha_est_n+/1, Gain3/1
  Sum/1 -> Integrator/1
  Sum1/1 -> Integrator1/1
  Gain5/1 -> Sum1/2
  Gain4/1 -> Sum/2
  Gain/1 -> Sum/1
  Gain3/1 -> Sum1/3

== system PLL_complete/MCCF PLL/MCCF module/Subsystem/Module 11- ==
  v_beta_n- : Inport
  n : Inport  Port=2
  v_alpha_n- : Inport  Port=3
  Gain{,3..5} (4 alike) : Gain  Gain=wc
  Integrator : Integrator
  Integrator1 : Integrator
  Product : Product  Inputs=3  RndMeth=Zero
  Product2 : Product  Inputs=3  RndMeth=Zero
  Sum : Sum  Inputs=-|+|+
  Sum1 : Sum  Inputs=-|+|-
  v_beta_est_n- : Outport
  v_alpha_est_n- : Outport  Port=2
  wires:
  Gain3/1 -> Sum1/3
  Gain/1 -> Sum/1
  Gain4/1 -> Sum/2
  Gain5/1 -> Sum1/2
  Sum1/1 -> Integrator1/1
  Sum/1 -> Integrator/1
  Integrator1/1 -> Gain3/1, v_alpha_est_n-/1, Product/3
  Integrator/1 -> Gain/1, v_beta_est_n-/1, Product2/3
  Product/1 -> Sum/3
  Product2/1 -> Sum1/1
  n/1 -> Product/1, Product2/1
  v_beta_n-/1 -> Gain4/1
  v_alpha_n-/1 -> Gain5/1
  [w_est_MCCF] -> Product/2, Product2/2

== system PLL_complete/MCCF PLL/MCCF module/Subsystem/Module 5+ ==
  v_beta_n+ : Inport
  n : Inport  Port=2
  v_alpha_n+ : Inport  Port=3
  Gain{,3..5} (4 alike) : Gain  Gain=wc
  Integrator : Integrator
  Integrator1 : Integrator
  Product : Product  Inputs=3  RndMeth=Zero
  Product2 : Product  Inputs=3  RndMeth=Zero
  Sum : Sum  Inputs=-|+|+
  Sum1 : Sum  Inputs=-|+|-
  v_beta_est_n+ : Outport
  v_alpha_est_n+ : Outport  Port=2
  wires:
  [w_est_MCCF] -> Product2/2, Product/2
  v_alpha_n+/1 -> Gain5/1
  v_beta_n+/1 -> Gain4/1
  n/1 -> Product2/1, Product/1
  Product2/1 -> Sum1/1
  Product/1 -> Sum/3
  Integrator/1 -> Product2/3, v_beta_est_n+/1, Gain/1
  Integrator1/1 -> Product/3, v_alpha_est_n+/1, Gain3/1
  Sum/1 -> Integrator/1
  Sum1/1 -> Integrator1/1
  Gain5/1 -> Sum1/2
  Gain4/1 -> Sum/2
  Gain/1 -> Sum/1
  Gain3/1 -> Sum1/3

== system PLL_complete/MCCF PLL/MCCF module/Subsystem/Module 5- ==
  v_beta_n- : Inport
  n : Inport  Port=2
  v_alpha_n- : Inport  Port=3
  Gain{,3..5} (4 alike) : Gain  Gain=wc
  Integrator : Integrator
  Integrator1 : Integrator
  Product : Product  Inputs=3  RndMeth=Zero
  Product2 : Product  Inputs=3  RndMeth=Zero
  Sum : Sum  Inputs=-|+|+
  Sum1 : Sum  Inputs=-|+|-
  v_beta_est_n- : Outport
  v_alpha_est_n- : Outport  Port=2
  wires:
  Gain3/1 -> Sum1/3
  Gain/1 -> Sum/1
  Gain4/1 -> Sum/2
  Gain5/1 -> Sum1/2
  Sum1/1 -> Integrator1/1
  Sum/1 -> Integrator/1
  Integrator1/1 -> Gain3/1, v_alpha_est_n-/1, Product/3
  Integrator/1 -> Gain/1, v_beta_est_n-/1, Product2/3
  Product/1 -> Sum/3
  Product2/1 -> Sum1/1
  n/1 -> Product/1, Product2/1
  v_beta_n-/1 -> Gain4/1
  v_alpha_n-/1 -> Gain5/1
  [w_est_MCCF] -> Product/2, Product2/2

== system PLL_complete/MCCF PLL/MCCF module/Subsystem/Module 7+ ==
  v_beta_n+ : Inport
  n : Inport  Port=2
  v_alpha_n+ : Inport  Port=3
  Gain{,3..5} (4 alike) : Gain  Gain=wc
  Integrator : Integrator
  Integrator1 : Integrator
  Product : Product  Inputs=3  RndMeth=Zero
  Product2 : Product  Inputs=3  RndMeth=Zero
  Sum : Sum  Inputs=-|+|+
  Sum1 : Sum  Inputs=-|+|-
  v_beta_est_n+ : Outport
  v_alpha_est_n+ : Outport  Port=2
  wires:
  Gain3/1 -> Sum1/3
  Gain/1 -> Sum/1
  Gain4/1 -> Sum/2
  Gain5/1 -> Sum1/2
  Sum1/1 -> Integrator1/1
  Sum/1 -> Integrator/1
  Integrator1/1 -> Gain3/1, v_alpha_est_n+/1, Product/3
  Integrator/1 -> Gain/1, v_beta_est_n+/1, Product2/3
  Product/1 -> Sum/3
  Product2/1 -> Sum1/1
  n/1 -> Product/1, Product2/1
  v_beta_n+/1 -> Gain4/1
  v_alpha_n+/1 -> Gain5/1
  [w_est_MCCF] -> Product/2, Product2/2

== system PLL_complete/MCCF PLL/MCCF module/Subsystem/Module 7- ==
  v_beta_n- : Inport
  n : Inport  Port=2
  v_alpha_n- : Inport  Port=3
  Gain{,3..5} (4 alike) : Gain  Gain=wc
  Integrator : Integrator
  Integrator1 : Integrator
  Product : Product  Inputs=3  RndMeth=Zero
  Product2 : Product  Inputs=3  RndMeth=Zero
  Sum : Sum  Inputs=-|+|+
  Sum1 : Sum  Inputs=-|+|-
  v_beta_est_n- : Outport
  v_alpha_est_n- : Outport  Port=2
  wires:
  [w_est_MCCF] -> Product2/2, Product/2
  v_alpha_n-/1 -> Gain5/1
  v_beta_n-/1 -> Gain4/1
  n/1 -> Product2/1, Product/1
  Product2/1 -> Sum1/1
  Product/1 -> Sum/3
  Integrator/1 -> Product2/3, v_beta_est_n-/1, Gain/1
  Integrator1/1 -> Product/3, v_alpha_est_n-/1, Gain3/1
  Sum/1 -> Integrator/1
  Sum1/1 -> Integrator1/1
  Gain5/1 -> Sum1/2
  Gain4/1 -> Sum/2
  Gain/1 -> Sum/1
  Gain3/1 -> Sum1/3
